simulink library "camera_update_lib"  (R2016b)
settings: Solver=ode45  StartTime=0.0  StopTime=10.0  RelTol=1e-3  EnableMultiTasking=on
undefined symbols (not defined in the file): accel_bias, ase_aug_state_bitmask, ase_hr_distance_r, ase_hr_r_mag, ase_local_mode_docking, ase_local_mode_map, ase_local_mode_perching, ase_minumum_resid_thresh, ase_ml_num_features, ase_of_num_aug, ase_of_num_features, ase_status_converged, ase_total_num_states, gyro_bias, hr_P_hr_ISS_ISS, hr_quat_ISS2hr, kfl_status, ml_mahal_distance, ml_P_cam_ISS_ISS, ml_quat_ISS2cam, of_mahal_distance, of_P_cam_ISS_ISS, of_quat_ISS2cam, P_EST_ISS_ISS, quat_ISS2B, tun_abp_q_body2dockcam, tun_abp_q_body2navcam, tun_abp_q_body2perchcam, tun_ase_dock_r_mag, tun_ase_dockcam_distortion, tun_ase_dockcam_inv_focal_length, tun_ase_enable_of, tun_ase_mahal_distance_max, tun_ase_map_error, tun_ase_min_hr_meas, tun_ase_min_ml_meas, tun_ase_min_of_meas, tun_ase_ml_forward_projection_time, tun_ase_navcam_distortion, tun_ase_navcam_inv_focal_length, tun_ase_of_r_mag, tun_ase_vis_r_mag, tun_ase_vocam_inv_focal_length, update_ML_features_cnt, update_OF_tracks_cnt, V_B_ISS_ISS
libraries: simulink x13, camera_update_lib x1
(part 1 of 2)
settings Model: Creator=jfusco1  LastModifiedBy=jfusco1
settings DataIOCC: LimitDataPoints=on  SaveFormat=Array
settings OptimizationCC: LifeSpan=inf
settings DebuggingCC: AllowSymbolicDim=off  SFUnexpectedBacktrackingDiag=warning  SFNoUnconditionalDefaultTransitionDiag=warning  SFExecutionAtInitializationDiag=none
settings HardwareCC: ProdBitPerPointer=32  ProdBitPerSizeT=32  ProdBitPerPtrDiffT=32  ProdLargestAtomicFloat=None  ProdIntDivRoundTo=Undefined  ProdEndianess=Unspecified  ProdWordSize=32  ProdHWDeviceType=32-bit Generic
settings ModelReferenceCC: PropagateSignalLabelsOutOfModel=off
settings GRTTargetCC: TargetLangStandard=C89/C90 (ANSI)  GeneratePreprocessorConditionals=Disable all
settings ConfigComp: CovMetricSettings=dw  CovHtmlReporting=on  CovSaveCumulativeToWorkspaceVar=on  CovSaveSingleToWorkspaceVar=on  CovExternalEMLEnable=off

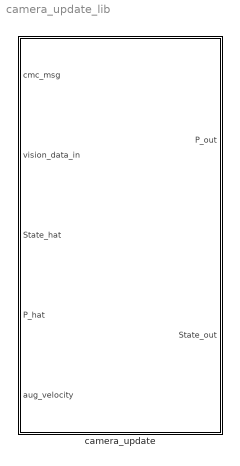
== system camera_update_lib ==
  camera_update : Subsystem

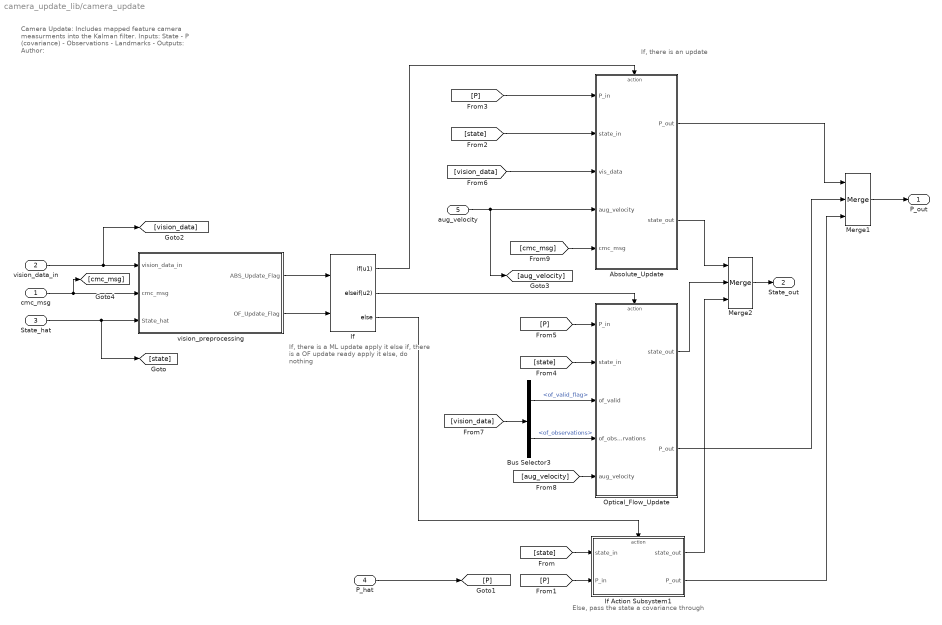
== system camera_update_lib/camera_update ==
  note: Camera Update:
      | Includes mapped feature camera measurments into the Kalman filter.
      |
      | Inputs:
      | State -
      | P (covariance) -
      | Observations -
      | Landmarks -
      |
      | Outputs:
      |
      | Author:
  note: If, there is an update
  note: Else, pass the state a covariance through
  note: If, there is a ML update apply it
      | else if, there is a OF update ready apply it
      | else, do nothing
  cmc_msg : Inport
  vision_data_in : Inport  Port=2
  State_hat : Inport  Port=3
  P_hat : Inport  Port=4  OutDataTypeStr=ase_cov_datatype
  aug_velocity : Inport  Port=5
  Absolute_Update : Subsystem  TreatAsAtomicUnit=on
  Bus Selector3 : BusSelector  OutputSignals=of_valid_flag,of_observations
  If : If  NumInputs=2  IfExpression=u1  ElseIfExpressions=u2
  If Action Subsystem1 : Subsystem  TreatAsAtomicUnit=on
  Merge1 : Merge  Inputs=3
  Merge2 : Merge  Inputs=3
  Optical_Flow_Update : Subsystem  TreatAsAtomicUnit=on
  vision_preprocessing : Subsystem
  P_out : Outport
  State_out : Outport  Port=2
  wires:
  cmc_msg/1 -> vision_preprocessing/2(cmc_msg), [cmc_msg]
  [aug_velocity] -> Optical_Flow_Update/5(aug_velocity)
  aug_velocity/1 -> Absolute_Update/4(aug_velocity), [aug_velocity]
  If/1 -> Absolute_Update/Action
  If/3 -> If Action Subsystem1/Action
  [P] -> If Action Subsystem1/2(P_in)
  [state] -> If Action Subsystem1/1(state_in)
  P_hat/1 -> [P]
  [state] -> Absolute_Update/2(state_in)
  [P] -> Absolute_Update/1(P_in)
  Absolute_Update/1(P_out) -> Merge1/1
  Merge1/1 -> P_out/1
  If Action Subsystem1/2(P_out) -> Merge1/3
  Merge2/1 -> State_out/1
  Absolute_Update/2(state_out) -> Merge2/1
  If Action Subsystem1/1(state_out) -> Merge2/3
  If/2 -> Optical_Flow_Update/Action
  [P] -> Optical_Flow_Update/1(P_in)
  [state] -> Optical_Flow_Update/2(state_in)
  [vision_data] -> Bus Selector3/1
  Bus Selector3/2 -> Optical_Flow_Update/4(of_observations)  "<of_observations>"
  Bus Selector3/1 -> Optical_Flow_Update/3(of_valid)  "<of_valid_flag>"
  Optical_Flow_Update/2(P_out) -> Merge1/2
  Optical_Flow_Update/1(state_out) -> Merge2/2
  vision_preprocessing/1("ABS_Update_Flag ") -> If/1
  vision_preprocessing/2(OF_Update_Flag) -> If/2
  State_hat/1 -> [state], vision_preprocessing/3(State_hat)
  vision_data_in/1 -> [vision_data], vision_preprocessing/1(vision_data_in)
  [vision_data] -> Absolute_Update/3(vis_data)
  [cmc_msg] -> Absolute_Update/5(cmc_msg)

== system camera_update_lib/camera_update/Absolute_Update ==
  P_in : Inport
  state_in : Inport  Port=2
  vis_data : Inport  Port=3
  aug_velocity : Inport  Port=4
  cmc_msg : Inport  Port=5
  Action Port : ActionPort  PropagateVarSize=During execution
  ML Update : Subsystem
  P_out : Outport
  state_out : Outport  Port=2
  wires:
  aug_velocity/1 -> ML Update/4(aug_velocity)
  state_in/1 -> ML Update/1(state_in)
  vis_data/1 -> ML Update/2(vis_data)
  P_in/1 -> ML Update/3(P_in)
  ML Update/1(State_out) -> state_out/1
  ML Update/2(P_out) -> P_out/1
  cmc_msg/1 -> ML Update/5(cmc_msg)

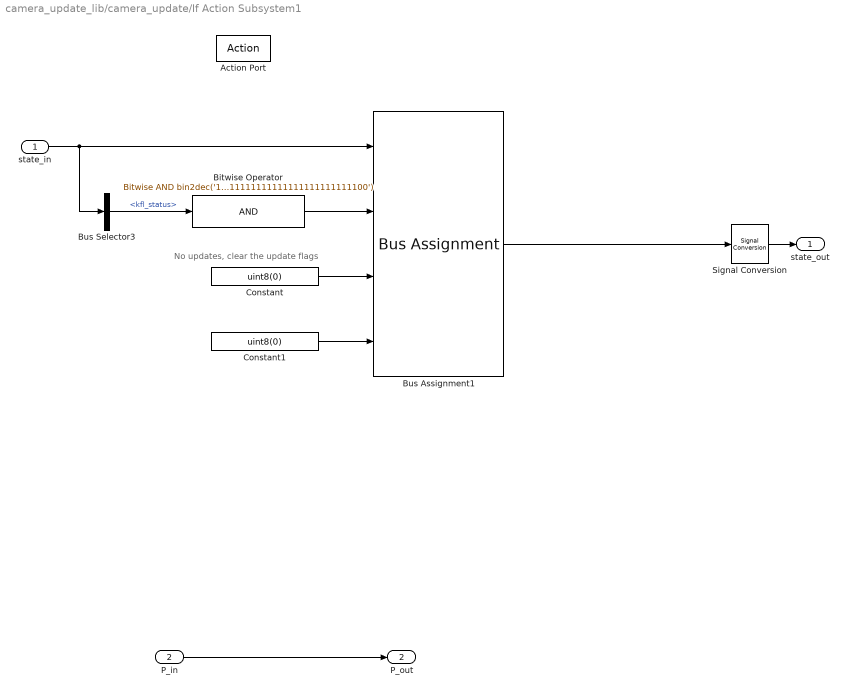
== system camera_update_lib/camera_update/If Action Subsystem1 ==
  note: No updates, clear the update flags
  state_in : Inport
  P_in : Inport  Port=2
  Action Port : ActionPort
  Bitwise Operator : simulink/Logic and Bit Operations/Bitwise Operator  logicop=AND  UseBitMask=on  BitMask=bin2dec('11111111111111111111111111111100')  BitMaskRealWorld=Stored Integer
  Bus Assignment1 : BusAssignment  AssignedSignals=kfl_status,update_OF_tracks_cnt,update_ML_features_cnt
  Bus Selector3 : BusSelector  OutputSignals=kfl_status
  Constant : Constant  Value=uint8(0)
  Constant1 : Constant  Value=uint8(0)
  Signal Conversion : SignalConversion  OverrideOpt=off
  state_out : Outport
  P_out : Outport  Port=2
  wires:
  Signal Conversion/1 -> state_out/1
  P_in/1 -> P_out/1
  Bus Selector3/1 -> Bitwise Operator/1  "<kfl_status>"
  Bitwise Operator/1 -> Bus Assignment1/2
  Bus Assignment1/1 -> Signal Conversion/1
  state_in/1 -> Bus Selector3/1, Bus Assignment1/1
  Constant/1 -> Bus Assignment1/3
  Constant1/1 -> Bus Assignment1/4

== system camera_update_lib/camera_update/Optical_Flow_Update ==
  P_in : Inport
  state_in : Inport  Port=2
  of_valid : Inport  Port=3
  of_observations : Inport  Port=4
  aug_velocity : Inport  Port=5
  Action Port : ActionPort  PropagateVarSize=During execution
  OF Update : Subsystem
  state_out : Outport
  P_out : Outport  Port=2
  wires:
  aug_velocity/1 -> OF Update/5(aug_velocity)
  OF Update/2(P_out) -> P_out/1
  OF Update/1(State_out) -> state_out/1
  P_in/1 -> OF Update/4(P_in)
  of_observations/1 -> OF Update/3(of_observations)
  of_valid/1 -> OF Update/2(of_valid)
  state_in/1 -> OF Update/1(state_in)

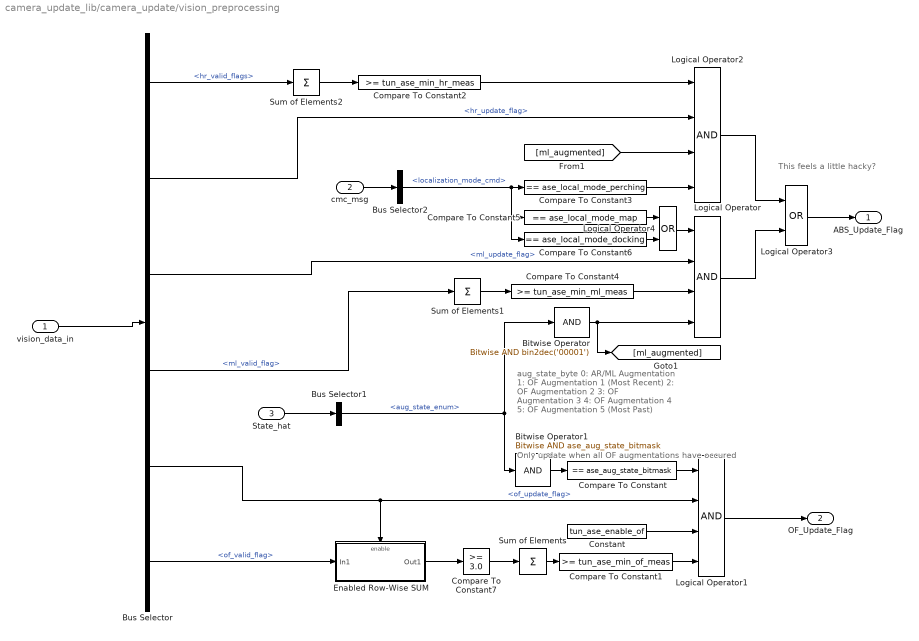
== system camera_update_lib/camera_update/vision_preprocessing ==
  note: This feels a little hacky?
  note: aug_state_byte
      | 0: AR/ML Augmentation
      | 1: OF Augmentation 1 (Most Recent)
      | 2: OF Augmentation 2
      | 3: OF Augmentation 3
      | 4: OF Augmentation 4
      | 5: OF Augmentation 5 (Most Past)
  note: Only update when all OF augmentations have occured
  vision_data_in : Inport
  cmc_msg : Inport  Port=2
  State_hat : Inport  Port=3
  Bitwise Operator : simulink/Logic and Bit Operations/Bitwise Operator  logicop=AND  UseBitMask=on  BitMask=bin2dec('00001')  BitMaskRealWorld=Stored Integer
  Bitwise Operator1 : simulink/Logic and Bit Operations/Bitwise Operator  logicop=AND  UseBitMask=on  BitMask=ase_aug_state_bitmask  BitMaskRealWorld=Stored Integer
  Bus Selector : BusSelector  OutputSignals=hr_valid_flags,hr_update_flag,ml_update_flag,ml_valid_flag,of_update_flag,of_valid_flag
  Bus Selector1 : BusSelector  OutputSignals=aug_state_enum
  Bus Selector2 : BusSelector  OutputSignals=localization_mode_cmd
  Compare To Constant : simulink/Logic and Bit Operations/Compare To Constant  relop===  const=ase_aug_state_bitmask  OutDataTypeStr=boolean
  Compare To Constant1 : simulink/Logic and Bit Operations/Compare To Constant  relop=>=  const=tun_ase_min_of_meas  OutDataTypeStr=boolean
  Compare To Constant2 : simulink/Logic and Bit Operations/Compare To Constant  relop=>=  const=tun_ase_min_hr_meas  OutDataTypeStr=boolean
  Compare To Constant3 : simulink/Logic and Bit Operations/Compare To Constant  relop===  const=ase_local_mode_perching  OutDataTypeStr=boolean
  Compare To Constant4 : simulink/Logic and Bit Operations/Compare To Constant  relop=>=  const=tun_ase_min_ml_meas  OutDataTypeStr=boolean
  Compare To Constant5 : simulink/Logic and Bit Operations/Compare To Constant  relop===  const=ase_local_mode_map  OutDataTypeStr=boolean
  Compare To Constant6 : simulink/Logic and Bit Operations/Compare To Constant  relop===  const=ase_local_mode_docking  OutDataTypeStr=boolean
  Compare To Constant7 : simulink/Logic and Bit Operations/Compare To Constant  relop=>=  const=3.0  OutDataTypeStr=boolean
  Constant : Constant  Value=tun_ase_enable_of
  Enabled Row-Wise SUM : Subsystem  TreatAsAtomicUnit=on
  Logical Operator : Logic  Inputs=4  AllPortsSameDT=off  OutDataTypeStr=boolean
  Logical Operator1 : Logic  Inputs=4  AllPortsSameDT=off  OutDataTypeStr=boolean
  Logical Operator2 : Logic  Inputs=4  AllPortsSameDT=off  OutDataTypeStr=boolean
  Logical Operator3 : Logic  Operator=OR  AllPortsSameDT=off  OutDataTypeStr=boolean
  Logical Operator4 : Logic  Operator=OR  AllPortsSameDT=off  OutDataTypeStr=boolean
  Sum of Elements : Sum  Inputs=+
  Sum of Elements1 : Sum  Inputs=+
  Sum of Elements2 : Sum  Inputs=+
  "ABS_Update_Flag " : Outport
  OF_Update_Flag : Outport  Port=2
  wires:
  Logical Operator3/1 -> "ABS_Update_Flag "/1
  Logical Operator/1 -> Logical Operator3/2
  Logical Operator2/1 -> Logical Operator3/1
  Bus Selector2/1 -> Compare To Constant3/1, Compare To Constant6/1, Compare To Constant5/1  "<localization_mode_cmd>"
  Compare To Constant3/1 -> Logical Operator2/4
  cmc_msg/1 -> Bus Selector2/1
  [ml_augmented] -> Logical Operator2/3
  Compare To Constant2/1 -> Logical Operator2/1
  Bus Selector/2 -> Logical Operator2/2  "<hr_update_flag>"
  Sum of Elements2/1 -> Compare To Constant2/1
  Bus Selector/1 -> Sum of Elements2/1  "<hr_valid_flags>"
  State_hat/1 -> Bus Selector1/1
  vision_data_in/1 -> Bus Selector/1
  Bus Selector/3 -> Logical Operator/2  "<ml_update_flag>"
  Bus Selector1/1 -> Bitwise Operator1/1, Bitwise Operator/1  "<aug_state_enum>"
  Bus Selector/5 -> Logical Operator1/2, Enabled Row-Wise SUM/Enable  "<of_update_flag>"
  Logical Operator1/1 -> OF_Update_Flag/1
  Constant/1 -> Logical Operator1/3
  Compare To Constant/1 -> Logical Operator1/1
  Bitwise Operator1/1 -> Compare To Constant/1
  Compare To Constant7/1 -> Sum of Elements/1
  Sum of Elements/1 -> Compare To Constant1/1
  Compare To Constant1/1 -> Logical Operator1/4
  Bitwise Operator/1 -> Logical Operator/4, [ml_augmented]
  Compare To Constant4/1 -> Logical Operator/3
  Sum of Elements1/1 -> Compare To Constant4/1
  Bus Selector/4 -> Sum of Elements1/1  "<ml_valid_flag>"
  Compare To Constant5/1 -> Logical Operator4/1
  Compare To Constant6/1 -> Logical Operator4/2
  Logical Operator4/1 -> Logical Operator/1
  Bus Selector/6 -> Enabled Row-Wise SUM/1(In1)  "<of_valid_flag>"
  Enabled Row-Wise SUM/1(Out1) -> Compare To Constant7/1

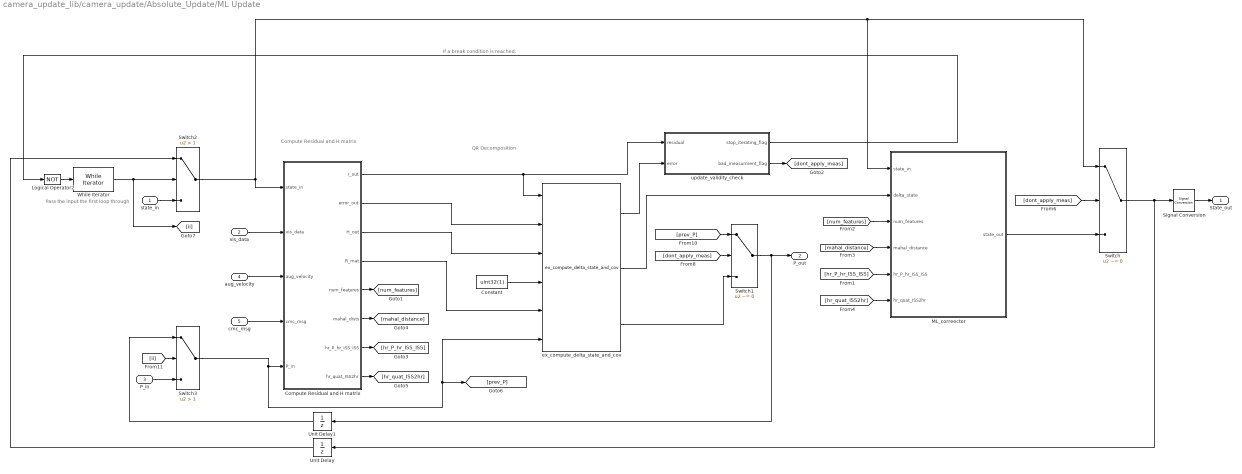
== system camera_update_lib/camera_update/Absolute_Update/ML Update ==
  note: Compute Residual and H matrix
  note: QR Decomposition
  note: Pass the input the first loop through
  note: If a break condition is reached.
  state_in : Inport
  vis_data : Inport  Port=2
  P_in : Inport  Port=3
  aug_velocity : Inport  Port=4
  cmc_msg : Inport  Port=5
  Compute Residual and H matrix : Subsystem
  Constant : Constant  Value=uint32(1)
  Logical Operator2 : Logic  Operator=NOT  Inputs=1  AllPortsSameDT=off  OutDataTypeStr=boolean
  ML_correector : Subsystem
  Signal Conversion : SignalConversion  OverrideOpt=off
  Switch : Switch  Criteria=u2 ~= 0
  Switch1 : Switch  Criteria=u2 ~= 0
  Switch2 : Switch  Criteria=u2 > Threshold  Threshold=1
  Switch3 : Switch  Criteria=u2 > Threshold  Threshold=1
  Unit Delay : UnitDelay  SampleTime=-1
  Unit Delay1 : UnitDelay  SampleTime=-1
  While Iterator : WhileIterator  MaxIters=ase_max_update_iterations  WhileBlockType=do-while  ResetStates=reset  ShowIterationPort=on
  ex_compute_delta_state_and_cov : S-Function  FunctionName=ex_compute_delta_state_and_cov  SFunctionDeploymentMode=off  EnableBusSupport=off  mask(Legacy Function){SFunctionSpec=int32 y1 = compute_delta_state_and_cov(single u1[], int32 u2, single u3[][], int32 size(u3, 1), int32 size(u3, 2),uint32 u4, single u5[][], single u6[][],single y2[size(u3, 2)], single y3[size(u3, 2)][size(u3, 2)]), ShowSpec=off}
      mask prompts: ShowSpec "Display function specification"
      mask help:
      | This block allows you to call the legacy functions specified by the following Legacy Code Tool definition:
      | def.SFunctionName = 'ex_compute_delta_state_and_cov';
      | def.OutputFcnSpec = 'int32 y1 = compute_delta_state_and_cov(single u1[], int32 u2, single u3[][], int32 size(u3, 1), int32 size(u3, 2),uint32 u4, single u5[][], single u6[][],single y2[size(u3, 2)], single y3[size(u3, 2)][size(u3, 2)])';
      | def.HeaderFiles = {'compute_delta_state_and_cov.h'};
      | def.SourceFiles = {'compute_delta_state_and_cov.cpp'};
      | def.IncPaths = {'cxx_functions/include', '/usr/include/eigen3'};
      | def.SrcPaths = {'cxx_functions/src', '/usr/include/eigen3/Eigen/src'};
      | def.Options.language = 'C++';
      mask Help: <p>This block was generated automatically by the Legacy Code Tool. For detailed help on this tool, call<a href="matlab:legacy_code('help')"> legacy_code('help')</a>.</p>
      mask Callback ShowSpec:
      | if strcmp(get_param(gcbh, 'ShowSpec'), 'on')
      |   set_param(gcbh, 'MaskDisplay', sprintf('fprintf(''%s'');', get_param(gcbh, 'SFunctionSpec')));
      | else
      |   set_param(gcbh, 'MaskDisplay', sprintf('fprintf(''%s'');', get_param(gcbh, 'FunctionName')));
      | end
      mask Display: fprintf('ex_compute_delta_state_and_cov');
  update_validity_check : Subsystem
  State_out : Outport
  P_out : Outport  Port=2
  wires:
  ex_compute_delta_state_and_cov/2 -> ML_correector/2(delta_state)
  ex_compute_delta_state_and_cov/3 -> Switch1/3
  Compute Residual and H matrix/3(H_out) -> ex_compute_delta_state_and_cov/3
  Compute Residual and H matrix/1(r_out) -> ex_compute_delta_state_and_cov/1, update_validity_check/1(residual)
  update_validity_check/2(bad_measurment_flag) -> [dont_apply_meas]
  [prev_P] -> Switch1/1
  Switch1/1 -> P_out/1, Unit Delay1/1
  [dont_apply_meas] -> Switch1/2
  Switch2/1 -> ML_correector/1(state_in), Switch/1, Compute Residual and H matrix/1(state_in)
  Switch/1 -> Unit Delay/1, Signal Conversion/1
  [dont_apply_meas] -> Switch/2
  Compute Residual and H matrix/4(R_mat) -> ex_compute_delta_state_and_cov/5
  Signal Conversion/1 -> State_out/1
  Switch3/1 -> Compute Residual and H matrix/5(P_in), ex_compute_delta_state_and_cov/6, [prev_P]
  state_in/1 -> Switch2/3
  Unit Delay/1 -> Switch2/1
  P_in/1 -> Switch3/3
  Unit Delay1/1 -> Switch3/1
  While Iterator/1 -> [ii], Switch2/2
  [ii] -> Switch3/2
  Logical Operator2/1 -> While Iterator/1
  update_validity_check/1(stop_iterating_flag) -> Logical Operator2/1
  ML_correector/1(state_out) -> Switch/3
  Compute Residual and H matrix/2(error_out) -> ex_compute_delta_state_and_cov/2
  Compute Residual and H matrix/5(num_features) -> [num_features]
  Compute Residual and H matrix/6(mahal_dists) -> [mahal_distance]
  vis_data/1 -> Compute Residual and H matrix/2(vis_data)
  ex_compute_delta_state_and_cov/1 -> update_validity_check/2(error)
  [num_features] -> ML_correector/3(num_features)
  [mahal_distance] -> ML_correector/4(mahal_distance)
  aug_velocity/1 -> Compute Residual and H matrix/3(aug_velocity)
  cmc_msg/1 -> Compute Residual and H matrix/4(cmc_msg)
  [hr_quat_ISS2hr] -> ML_correector/6(hr_quat_ISS2hr)
  [hr_P_hr_ISS_ISS] -> ML_correector/5(hr_P_hr_ISS_ISS)
  Compute Residual and H matrix/7(hr_P_hr_ISS_ISS) -> [hr_P_hr_ISS_ISS]
  Compute Residual and H matrix/8(hr_quat_ISS2hr) -> [hr_quat_ISS2hr]
  Constant/1 -> ex_compute_delta_state_and_cov/4

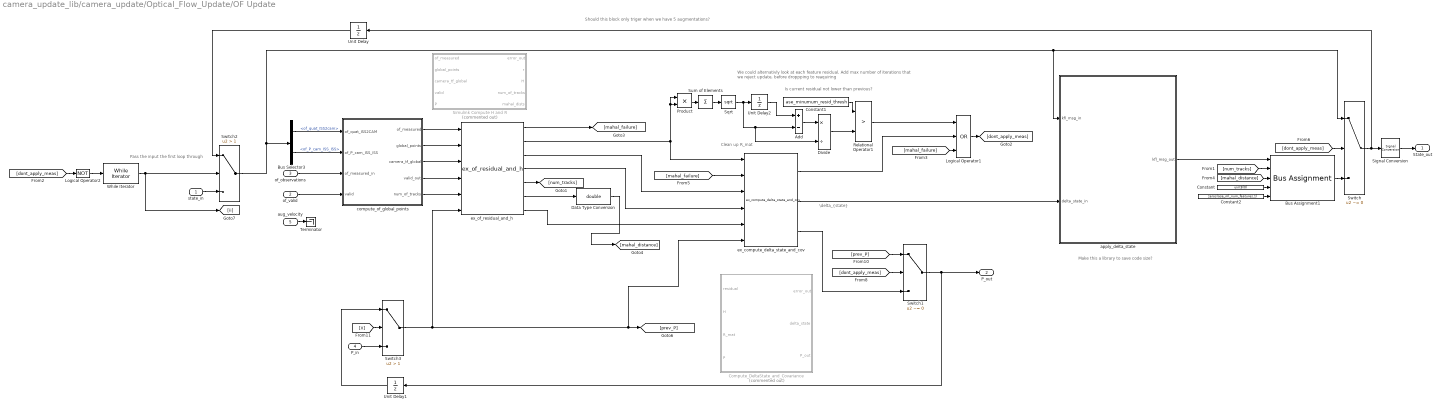
== system camera_update_lib/camera_update/Optical_Flow_Update/OF Update ==
  note: Clean up R_mat
  note: Pass the input the first loop through
  note: \delta_{state}
  note: Make this a library to save code size?
  note: Should this block only triger when we have 5 augmentations?
  note: Is current residual not lower than previous?
  note: We could alternativly look at each feature residual.
      | Add max number of iterations that we reject update, before droppping to reaquiring
  state_in : Inport
  of_valid : Inport  Port=2
  of_observations : Inport  Port=3
  P_in : Inport  Port=4  PortDimensions=[ase_total_num_states ase_total_num_states]
  aug_velocity : Inport  Port=5
  Add : Sum  Inputs=+-
  Bus Assignment1 : BusAssignment  AssignedSignals=update_OF_tracks_cnt,of_mahal_distance,update_ML_features_cnt,ml_mahal_distance
  Bus Selector3 : BusSelector  OutputSignals=of_quat_ISS2cam,of_P_cam_ISS_ISS
  Compute_DeltaState_and_Covariance : MATLAB Function  Commented=on  TreatAsAtomicUnit=on
  Constant : Constant  Value=uint8(0)
  Constant1 : Constant  Value=ase_minumum_resid_thresh
  Constant2 : Constant  Value=zeros(ase_ml_num_features,1)
  Data Type Conversion : DataTypeConversion  OutDataTypeStr=double
  Divide : Product  Inputs=*/
  Logical Operator1 : Logic  Operator=OR  Inputs=3  AllPortsSameDT=off  OutDataTypeStr=boolean
  Logical Operator2 : Logic  Operator=NOT  Inputs=1  AllPortsSameDT=off  OutDataTypeStr=boolean
  Product : Product
  Relational Operator1 : RelationalOperator  Operator=>  OutDataTypeStr=boolean  RndMeth=Nearest
  Signal Conversion : SignalConversion  OverrideOpt=off
  Simulink Compute H and R : Subsystem  Commented=on  TreatAsAtomicUnit=on
  Sqrt : Sqrt  SaturateOnIntegerOverflow=on
  Sum of Elements : Sum  Inputs=+
  Switch : Switch  Criteria=u2 ~= 0
  Switch1 : Switch  Criteria=u2 ~= 0
  Switch2 : Switch  Criteria=u2 > Threshold  Threshold=1
  Switch3 : Switch  Criteria=u2 > Threshold  Threshold=1
  Terminator : Terminator
  Unit Delay : UnitDelay  SampleTime=-1
  Unit Delay1 : UnitDelay  SampleTime=-1
  Unit Delay2 : UnitDelay  InitialCondition=inf  SampleTime=-1
      settings: AttributesFormatString=IC: %<InitialCondition>
  While Iterator : WhileIterator  MaxIters=ase_max_of_update_iterations  WhileBlockType=do-while  ResetStates=reset  ShowIterationPort=on
  apply_delta_state : Subsystem
  compute_of_global_points : MATLAB Function  TreatAsAtomicUnit=on
  ex_compute_delta_state_and_cov : S-Function  FunctionName=ex_compute_delta_state_and_cov  SFunctionDeploymentMode=off  EnableBusSupport=off  mask(Legacy Function){SFunctionSpec=int32 y1 = compute_delta_state_and_cov(single u1[], int32 u2, single u3[][], int32 size(u3, 1), int32 size(u3, 2),uint32 u4, single u5[][], single u6[][],single y2[size(u3, 2)], single y3[size(u3, 2)][size(u3, 2)]), ShowSpec=off}
      mask prompts: ShowSpec "Display function specification"
      mask help:
      | This block allows you to call the legacy functions specified by the following Legacy Code Tool definition:
      | def.SFunctionName = 'ex_compute_delta_state_and_cov';
      | def.OutputFcnSpec = 'int32 y1 = compute_delta_state_and_cov(single u1[], int32 u2, single u3[][], int32 size(u3, 1), int32 size(u3, 2),uint32 u4, single u5[][], single u6[][],single y2[size(u3, 2)], single y3[size(u3, 2)][size(u3, 2)])';
      | def.HeaderFiles = {'compute_delta_state_and_cov.h'};
      | def.SourceFiles = {'compute_delta_state_and_cov.cpp'};
      | def.IncPaths = {'cxx_functions/include', '/usr/include/eigen3'};
      | def.SrcPaths = {'cxx_functions/src', '/usr/include/eigen3/Eigen/src'};
      | def.Options.language = 'C++';
      mask Help: <p>This block was generated automatically by the Legacy Code Tool. For detailed help on this tool, call<a href="matlab:legacy_code('help')"> legacy_code('help')</a>.</p>
      mask Callback ShowSpec:
      | if strcmp(get_param(gcbh, 'ShowSpec'), 'on')
      |   set_param(gcbh, 'MaskDisplay', sprintf('fprintf(''%s'');', get_param(gcbh, 'SFunctionSpec')));
      | else
      |   set_param(gcbh, 'MaskDisplay', sprintf('fprintf(''%s'');', get_param(gcbh, 'FunctionName')));
      | end
      mask Display: fprintf('ex_compute_delta_state_and_cov');
  ex_of_residual_and_h : S-Function  FunctionName=ex_of_residual_and_h  Parameters=SParameter1, SParameter2, SParameter3, SParameter4, SParameter5, SParameter6  SFunctionDeploymentMode=off  EnableBusSupport=off  mask(Legacy Function){SFunctionSpec=int32 y1 = of_residual_and_h(single u1[1600], single u2[4][50], single u3[64][4], int32 u4[50][16], int32 u5, int32 p1, int32 p2, single p3, single p4, single p5, single p6, single u6[117][117], single y2[96], single y3[96][117], uint32 y4[1], uint8 y5[1], single y6[50], single y7[96][96]), SParameter1=ase_of_num_aug, SParameter2=ase_of_num_features, SParameter3=tun_ase_mahal_distance_max, SParameter4=tun_ase_of_r_mag, SParameter5=tun_ase_navcam_inv_focal_length, SParameter6=tun_ase_navcam_distortion, ShowSpec=off}
      mask prompts: SParameter1 "P1:"; SParameter2 "P2:"; SParameter3 "P3:"; SParameter4 "P4:"; SParameter5 "P5:"; SParameter6 "P6:"; ShowSpec "Display function specification"
      mask help:
      | This block allows you to call the legacy functions specified by the following Legacy Code Tool definition:
      | def.SFunctionName = 'ex_of_residual_and_h';
      | def.OutputFcnSpec = 'int32 y1 = of_residual_and_h(single u1[1600], single u2[4][50], single u3[64][4], int32 u4[50][16], int32 u5, int32 p1, int32 p2, single p3, single p4, single p5, single p6, single u6[117][117], single y2[96], single y3[96][117], uint32 y4[1], uint8 y5[1], single y6[50], single y7[96][96])';
      | def.HeaderFiles = {'of_residual_and_h.h'};
      | def.SourceFiles = {'of_residual_and_h.cpp'};
      | def.IncPaths = {'./cxx_functions/include', '/usr/include/eigen3/'};
      | def.SrcPaths = {'./cxx_functions/src', '/usr/include/eigen3/Eigen/src'};
      | def.Options.language = 'C++';
      | def.Options.supportsMultipleExecInstances = true;
      mask Help: <p>This block was generated automatically by the Legacy Code Tool. For detailed help on this tool, call<a href="matlab:legacy_code('help')"> legacy_code('help')</a>.</p>
      mask Callback ShowSpec:
      | if strcmp(get_param(gcbh, 'ShowSpec'), 'on')
      |   set_param(gcbh, 'MaskDisplay', sprintf('fprintf(''%s'');', get_param(gcbh, 'SFunctionSpec')));
      | else
      |   set_param(gcbh, 'MaskDisplay', sprintf('fprintf(''%s'');', get_param(gcbh, 'FunctionName')));
      | end
      mask Display: fprintf('ex_of_residual_and_h');
  State_out : Outport
  P_out : Outport  Port=2
  wires:
  Constant2/1 -> Bus Assignment1/5
  Constant/1 -> Bus Assignment1/4
  [mahal_distance] -> Bus Assignment1/3
  Logical Operator2/1 -> While Iterator/1
  [ii] -> Switch3/2
  While Iterator/1 -> Switch2/2, [ii]
  Unit Delay1/1 -> Switch3/1
  P_in/1 -> Switch3/3
  Unit Delay/1 -> Switch2/1
  state_in/1 -> Switch2/3
  Switch3/1 -> ex_of_residual_and_h/6, ex_compute_delta_state_and_cov/6, [prev_P]
  Signal Conversion/1 -> State_out/1
  [dont_apply_meas] -> Switch/2
  Switch/1 -> Unit Delay/1, Signal Conversion/1
  Switch2/1 -> apply_delta_state/1(kfl_msg_in), Switch/1, Bus Selector3/1
  [dont_apply_meas] -> Switch1/2
  Switch1/1 -> P_out/1, Unit Delay1/1
  [prev_P] -> Switch1/1
  Bus Selector3/1 -> compute_of_global_points/1(of_quat_ISS2CAM)  "<of_quat_ISS2cam>"
  Bus Selector3/2 -> compute_of_global_points/2(of_P_cam_ISS_ISS)  "<of_P_cam_ISS_ISS>"
  of_valid/1 -> compute_of_global_points/4(valid)
  of_observations/1 -> compute_of_global_points/3(of_measured_in)
  [num_tracks] -> Bus Assignment1/2
  Bus Assignment1/1 -> Switch/3
  aug_velocity/1 -> Terminator/1
  Constant1/1 -> Relational Operator1/1
  Divide/1 -> Relational Operator1/2
  Add/1 -> Divide/1
  Product/1 -> Sum of Elements/1
  Unit Delay2/1 -> Add/1
  ex_of_residual_and_h/2 -> ex_compute_delta_state_and_cov/1, Product/1, Product/2
  Sqrt/1 -> Divide/2, Add/2, Unit Delay2/1
  Logical Operator1/1 -> [dont_apply_meas]
  Relational Operator1/1 -> Logical Operator1/1
  [dont_apply_meas] -> Logical Operator2/1
  ex_of_residual_and_h/1 -> [mahal_failure]
  ex_of_residual_and_h/5 -> [num_tracks]
  Data Type Conversion/1 -> [mahal_distance]
  ex_of_residual_and_h/6 -> Data Type Conversion/1
  compute_of_global_points/5(num_of_tracks) -> ex_of_residual_and_h/5
  compute_of_global_points/4(valid_out) -> ex_of_residual_and_h/4
  compute_of_global_points/3(camera_tf_global) -> ex_of_residual_and_h/3
  compute_of_global_points/2(global_points) -> ex_of_residual_and_h/2
  compute_of_global_points/1(of_measured) -> ex_of_residual_and_h/1
  [mahal_failure] -> ex_compute_delta_state_and_cov/2
  ex_compute_delta_state_and_cov/1 -> Logical Operator1/2
  ex_compute_delta_state_and_cov/2 -> apply_delta_state/2(delta_state_in)
  ex_compute_delta_state_and_cov/3 -> Switch1/3
  ex_of_residual_and_h/3 -> ex_compute_delta_state_and_cov/3
  ex_of_residual_and_h/4 -> ex_compute_delta_state_and_cov/4
  Sum of Elements/1 -> Sqrt/1
  [mahal_failure] -> Logical Operator1/3
  apply_delta_state/1(kfl_msg_out) -> Bus Assignment1/1
  ex_of_residual_and_h/7 -> ex_compute_delta_state_and_cov/5

== system camera_update_lib/camera_update/vision_preprocessing/Enabled Row-Wise SUM ==
  In1 : Inport
  Enable : EnablePort
  Sum of Elements3 : Sum  Inputs=+  CollapseMode=Specified dimension  CollapseDim=2
  Out1 : Outport
  wires:
  In1/1 -> Sum of Elements3/1
  Sum of Elements3/1 -> Out1/1

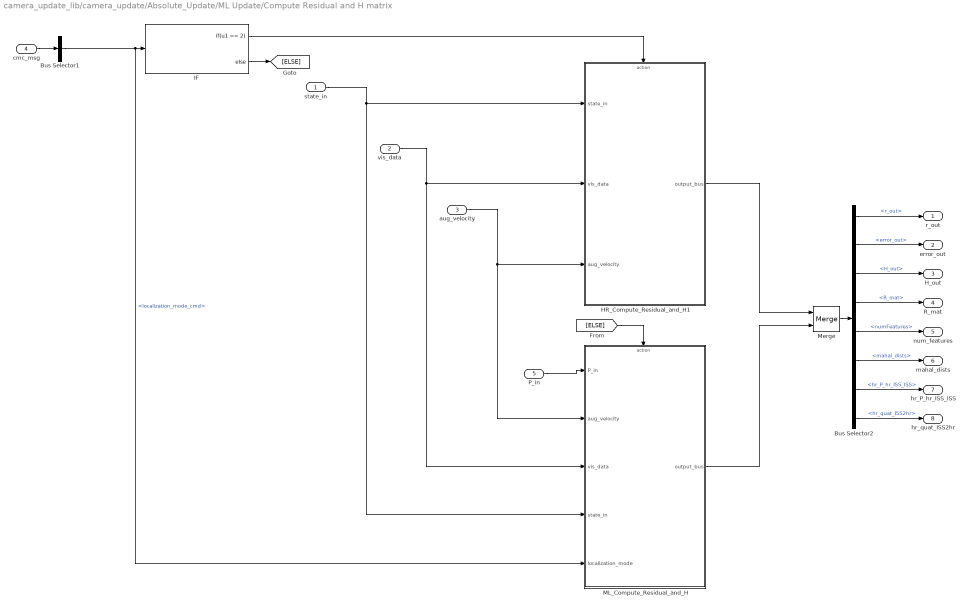
== system camera_update_lib/camera_update/Absolute_Update/ML Update/Compute Residual and H matrix ==
  state_in : Inport
  vis_data : Inport  Port=2
  aug_velocity : Inport  Port=3
  cmc_msg : Inport  Port=4
  P_in : Inport  Port=5
  Bus Selector1 : BusSelector  OutputSignals=localization_mode_cmd
  Bus Selector2 : BusSelector  OutputSignals=r_out,error_out,H_out,R_mat,numFeatures,mahal_dists,hr_P_hr_ISS_ISS,hr_quat_ISS2hr
  HR_Compute_Residual_and_H1 : Subsystem  TreatAsAtomicUnit=on
  IF : If  IfExpression=u1 == 2
  ML_Compute_Residual_and_H : Subsystem  TreatAsAtomicUnit=on
  Merge : Merge
  r_out : Outport
  error_out : Outport  Port=2
  H_out : Outport  Port=3
  R_mat : Outport  Port=4
  num_features : Outport  Port=5
  mahal_dists : Outport  Port=6
  hr_P_hr_ISS_ISS : Outport  Port=7
  hr_quat_ISS2hr : Outport  Port=8
  wires:
  IF/1 -> HR_Compute_Residual_and_H1/Action
  state_in/1 -> ML_Compute_Residual_and_H/4(state_in), HR_Compute_Residual_and_H1/1(state_in)
  vis_data/1 -> ML_Compute_Residual_and_H/3(vis_data), HR_Compute_Residual_and_H1/2(vis_data)
  P_in/1 -> ML_Compute_Residual_and_H/1(P_in)
  aug_velocity/1 -> ML_Compute_Residual_and_H/2(aug_velocity), HR_Compute_Residual_and_H1/3(aug_velocity)
  IF/2 -> [ELSE]
  [ELSE] -> ML_Compute_Residual_and_H/Action
  Merge/1 -> Bus Selector2/1
  Bus Selector2/1 -> r_out/1  "<r_out>"
  Bus Selector2/2 -> error_out/1  "<error_out>"
  Bus Selector2/3 -> H_out/1  "<H_out>"
  Bus Selector2/4 -> R_mat/1  "<R_mat>"
  Bus Selector2/5 -> num_features/1  "<numFeatures>"
  Bus Selector2/6 -> mahal_dists/1  "<mahal_dists>"
  HR_Compute_Residual_and_H1/1(output_bus) -> Merge/1
  ML_Compute_Residual_and_H/1(output_bus) -> Merge/2
  cmc_msg/1 -> Bus Selector1/1
  Bus Selector1/1 -> ML_Compute_Residual_and_H/5(localization_mode), IF/1  "<localization_mode_cmd>"
  Bus Selector2/7 -> hr_P_hr_ISS_ISS/1  "<hr_P_hr_ISS_ISS>"
  Bus Selector2/8 -> hr_quat_ISS2hr/1  "<hr_quat_ISS2hr>"

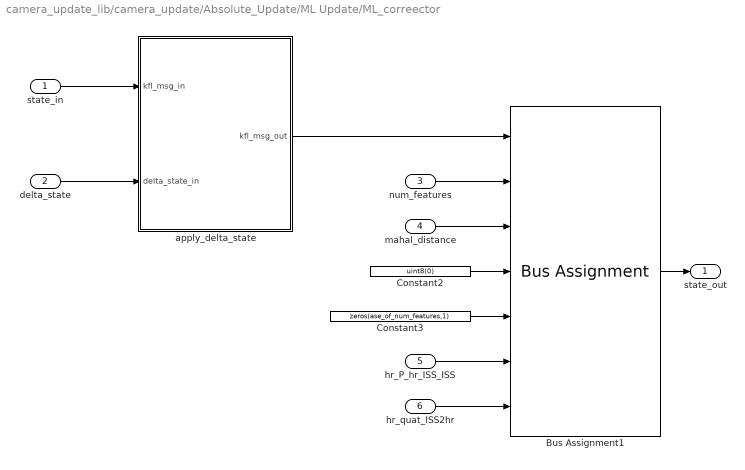
== system camera_update_lib/camera_update/Absolute_Update/ML Update/ML_correector ==
  state_in : Inport
  delta_state : Inport  Port=2
  num_features : Inport  Port=3
  mahal_distance : Inport  Port=4
  hr_P_hr_ISS_ISS : Inport  Port=5
  hr_quat_ISS2hr : Inport  Port=6
  Bus Assignment1 : BusAssignment  AssignedSignals=update_ML_features_cnt,ml_mahal_distance,update_OF_tracks_cnt,of_mahal_distance,hr_P_hr_ISS_ISS,hr_quat_ISS2hr
  Constant2 : Constant  Value=uint8(0)
  Constant3 : Constant  Value=zeros(ase_of_num_features,1)
  apply_delta_state : Subsystem
  state_out : Outport
  wires:
  mahal_distance/1 -> Bus Assignment1/3
  num_features/1 -> Bus Assignment1/2
  Constant2/1 -> Bus Assignment1/4
  Constant3/1 -> Bus Assignment1/5
  Bus Assignment1/1 -> state_out/1
  hr_quat_ISS2hr/1 -> Bus Assignment1/7
  hr_P_hr_ISS_ISS/1 -> Bus Assignment1/6
  apply_delta_state/1(kfl_msg_out) -> Bus Assignment1/1
  delta_state/1 -> apply_delta_state/2(delta_state_in)
  state_in/1 -> apply_delta_state/1(kfl_msg_in)

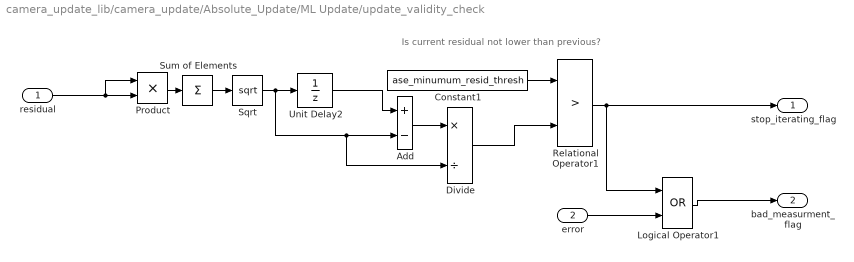
== system camera_update_lib/camera_update/Absolute_Update/ML Update/update_validity_check ==
  note: Is current residual not lower than previous?
  residual : Inport
  error : Inport  Port=2
  Add : Sum  Inputs=+-
  Constant1 : Constant  Value=ase_minumum_resid_thresh
  Divide : Product  Inputs=*/
  Logical Operator1 : Logic  Operator=OR  AllPortsSameDT=off  OutDataTypeStr=boolean
  Product : Product
  Relational Operator1 : RelationalOperator  Operator=>  OutDataTypeStr=boolean  RndMeth=Nearest
  Sqrt : Sqrt  SaturateOnIntegerOverflow=on
  Sum of Elements : Sum  Inputs=+
  Unit Delay2 : UnitDelay  InitialCondition=inf  SampleTime=-1
      settings: AttributesFormatString=IC: %<InitialCondition>
  stop_iterating_flag : Outport
  bad_measurment_flag : Outport  Port=2
  wires:
  residual/1 -> Product/2, Product/1
  Logical Operator1/1 -> bad_measurment_flag/1
  Unit Delay2/1 -> Add/1
  Product/1 -> Sum of Elements/1
  Sum of Elements/1 -> Sqrt/1
  Sqrt/1 -> Divide/2, Add/2, Unit Delay2/1
  Add/1 -> Divide/1
  Divide/1 -> Relational Operator1/2
  Constant1/1 -> Relational Operator1/1
  Relational Operator1/1 -> stop_iterating_flag/1, Logical Operator1/1
  error/1 -> Logical Operator1/2

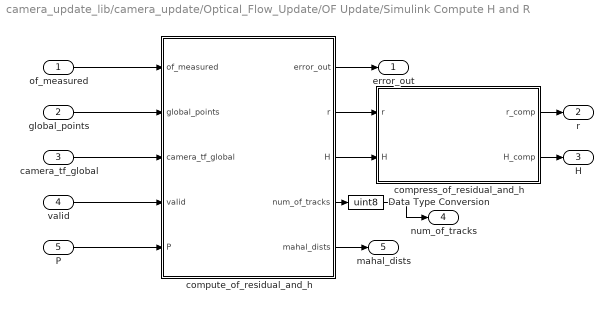
== system camera_update_lib/camera_update/Optical_Flow_Update/OF Update/Simulink Compute H and R ==
  of_measured : Inport
  global_points : Inport  Port=2
  camera_tf_global : Inport  Port=3
  valid : Inport  Port=4
  P : Inport  Port=5
  Data Type Conversion : DataTypeConversion  OutDataTypeStr=uint8
  compress_of_residual_and_h : MATLAB Function  TreatAsAtomicUnit=on
  compute_of_residual_and_h : MATLAB Function  TreatAsAtomicUnit=on
  error_out : Outport
  r : Outport  Port=2
  H : Outport  Port=3
  num_of_tracks : Outport  Port=4
  mahal_dists : Outport  Port=5
  wires:
  compute_of_residual_and_h/3(H) -> compress_of_residual_and_h/2(H)
  compute_of_residual_and_h/2(r) -> compress_of_residual_and_h/1(r)
  camera_tf_global/1 -> compute_of_residual_and_h/3(camera_tf_global)
  global_points/1 -> compute_of_residual_and_h/2(global_points)
  of_measured/1 -> compute_of_residual_and_h/1(of_measured)
  compress_of_residual_and_h/1(r_comp) -> r/1
  compute_of_residual_and_h/4(num_of_tracks) -> Data Type Conversion/1
  valid/1 -> compute_of_residual_and_h/4(valid)
  P/1 -> compute_of_residual_and_h/5(P)
  compress_of_residual_and_h/2(H_comp) -> H/1
  Data Type Conversion/1 -> num_of_tracks/1
  compute_of_residual_and_h/5(mahal_dists) -> mahal_dists/1
  compute_of_residual_and_h/1(error_out) -> error_out/1

== system camera_update_lib/camera_update/Optical_Flow_Update/OF Update/apply_delta_state ==
  kfl_msg_in : Inport
  delta_state_in : Inport  Port=2
  Bus Assignment1 : BusAssignment  AssignedSignals=quat_ISS2B,gyro_bias,V_B_ISS_ISS,accel_bias,P_EST_ISS_ISS,ml_quat_ISS2cam,ml_P_cam_ISS_ISS,kfl_status,of_quat_ISS2cam,of_P_cam_ISS_ISS
  Bus Selector1 : BusSelector  OutputSignals=quat_ISS2B,gyro_bias,V_B_ISS_ISS,accel_bias,P_EST_ISS_ISS,ml_quat_ISS2cam,ml_P_cam_ISS_ISS,kfl_status,of_quat_ISS2cam,of_P_cam_ISS_ISS
  Constant : Constant  Value=uint16(2)
  ex_apply_delta_state : camera_update_lib/camera_update/Absolute_Update/ML Update/ML_correector/apply_delta_state/ex_apply_delta_state  SFunctionSpec=void apply_delta_state(single u1[], int32 size(u1, 1), uint16 u2, single u3[4], single u4[3], single u5[3], single u6[3], single u7[3], single u8[4], single u9[3], uint16 u10, single u11[16][4], single u12[16][3], single y1[4], single y2[3], single y3[3], single y4[3], single y5[3], single y6[4], single y7[3], uint16 y8[1], single y9[16][4], single y10[16][3])  ShowSpec=off
  kfl_msg_out : Outport  OutDataTypeStr=Bus: kfl_msg
  wires:
  ex_apply_delta_state/10 -> Bus Assignment1/11
  ex_apply_delta_state/8 -> Bus Assignment1/9
  ex_apply_delta_state/7 -> Bus Assignment1/8
  ex_apply_delta_state/5 -> Bus Assignment1/6
  ex_apply_delta_state/4 -> Bus Assignment1/5
  ex_apply_delta_state/3 -> Bus Assignment1/4
  ex_apply_delta_state/2 -> Bus Assignment1/3
  Bus Selector1/10 -> ex_apply_delta_state/12  "<of_P_cam_ISS_ISS>"
  Bus Selector1/9 -> ex_apply_delta_state/11  "<of_quat_ISS2cam>"
  Bus Selector1/8 -> ex_apply_delta_state/10  "<kfl_status>"
  Bus Selector1/7 -> ex_apply_delta_state/9  "<ml_P_cam_ISS_ISS>"
  Bus Selector1/6 -> ex_apply_delta_state/8  "<ml_quat_ISS2cam>"
  Bus Selector1/5 -> ex_apply_delta_state/7  "<P_EST_ISS_ISS>"
  Bus Selector1/4 -> ex_apply_delta_state/6  "<accel_bias>"
  Bus Selector1/3 -> ex_apply_delta_state/5  "<V_B_ISS_ISS>"
  Bus Selector1/2 -> ex_apply_delta_state/4  "<gyro_bias>"
  Bus Selector1/1 -> ex_apply_delta_state/3  "<quat_ISS2B>"
  Constant/1 -> ex_apply_delta_state/2
  delta_state_in/1 -> ex_apply_delta_state/1
  kfl_msg_in/1 -> Bus Assignment1/1, Bus Selector1/1
  Bus Assignment1/1 -> kfl_msg_out/1
  ex_apply_delta_state/1 -> Bus Assignment1/2
  ex_apply_delta_state/9 -> Bus Assignment1/10
  ex_apply_delta_state/6 -> Bus Assignment1/7

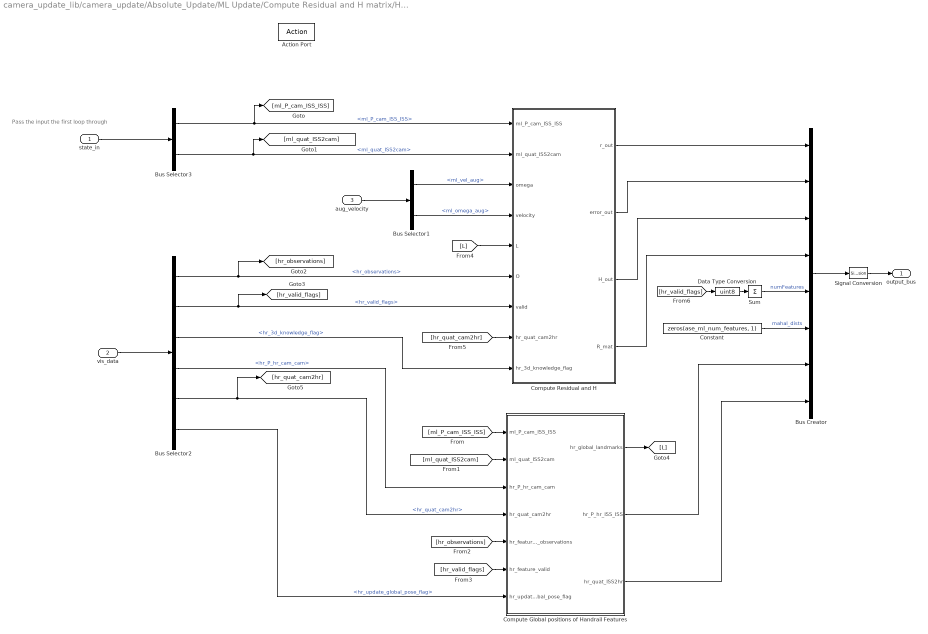
== system camera_update_lib/camera_update/Absolute_Update/ML Update/Compute Residual and H matrix/HR_Compute_Residual_and_H1 ==
  note: Pass the input the first loop through
  state_in : Inport
  vis_data : Inport  Port=2
  aug_velocity : Inport  Port=3
  Action Port : ActionPort
  Bus Creator : BusCreator  Inputs=8
  Bus Selector1 : BusSelector  OutputSignals=ml_vel_aug,ml_omega_aug
  Bus Selector2 : BusSelector  OutputSignals=hr_observations,hr_valid_flags,hr_3d_knowledge_flag,hr_P_hr_cam_cam,hr_quat_cam2hr,hr_update_global_pose_flag
  Bus Selector3 : BusSelector  OutputSignals=ml_P_cam_ISS_ISS,ml_quat_ISS2cam
  Compute Global positions of Handrail Features : MATLAB Function  TreatAsAtomicUnit=on
  Compute Residual and H : MATLAB Function  TreatAsAtomicUnit=on
  Constant : Constant  Value=zeros(ase_ml_num_features, 1)  VectorParams1D=off
  Data Type Conversion : DataTypeConversion  OutDataTypeStr=uint8
  Signal Conversion : SignalConversion  OverrideOpt=off
  Sum : Sum  Inputs=+
  output_bus : Outport
  wires:
  Sum/1 -> Bus Creator/5  "numFeatures"
  Constant/1 -> Bus Creator/6  "mahal_dists"
  Signal Conversion/1 -> output_bus/1
  Bus Creator/1 -> Signal Conversion/1
  Compute Residual and H/4(R_mat) -> Bus Creator/4
  Compute Residual and H/3(H_out) -> Bus Creator/3
  Compute Residual and H/2(error_out) -> Bus Creator/2
  Compute Residual and H/1(r_out) -> Bus Creator/1
  vis_data/1 -> Bus Selector2/1
  Bus Selector2/1 -> [hr_observations], Compute Residual and H/6(O)  "<hr_observations>"
  Bus Selector3/2 -> [ml_quat_ISS2cam], Compute Residual and H/2(ml_quat_ISS2cam)  "<ml_quat_ISS2cam>"
  Bus Selector3/1 -> [ml_P_cam_ISS_ISS], Compute Residual and H/1(ml_P_cam_ISS_ISS)  "<ml_P_cam_ISS_ISS>"
  state_in/1 -> Bus Selector3/1
  aug_velocity/1 -> Bus Selector1/1
  Bus Selector1/1 -> Compute Residual and H/3(omega)  "<ml_vel_aug>"
  Bus Selector1/2 -> Compute Residual and H/4(velocity)  "<ml_omega_aug>"
  Bus Selector2/3 -> Compute Residual and H/9(hr_3d_knowledge_flag)  "<hr_3d_knowledge_flag>"
  Bus Selector2/4 -> Compute Global positions of Handrail Features/3(hr_P_hr_cam_cam)  "<hr_P_hr_cam_cam>"
  Bus Selector2/5 -> Compute Global positions of Handrail Features/4(hr_quat_cam2hr), [hr_quat_cam2hr]  "<hr_quat_cam2hr>"
  Bus Selector2/6 -> Compute Global positions of Handrail Features/7(hr_update_global_pose_flag)  "<hr_update_global_pose_flag>"
  Compute Global positions of Handrail Features/2(hr_P_hr_ISS_ISS) -> Bus Creator/7
  Compute Global positions of Handrail Features/3(hr_quat_ISS2hr) -> Bus Creator/8
  [ml_P_cam_ISS_ISS] -> Compute Global positions of Handrail Features/1(ml_P_cam_ISS_ISS)
  [ml_quat_ISS2cam] -> Compute Global positions of Handrail Features/2(ml_quat_ISS2cam)
  Bus Selector2/2 -> [hr_valid_flags], Compute Residual and H/7(valid)  "<hr_valid_flags>"
  [hr_observations] -> Compute Global positions of Handrail Features/5(hr_feature_observations)
  [hr_valid_flags] -> Compute Global positions of Handrail Features/6(hr_feature_valid)
  Compute Global positions of Handrail Features/1(hr_global_landmarks) -> [L]
  [L] -> Compute Residual and H/5(L)
  [hr_quat_cam2hr] -> Compute Residual and H/8(hr_quat_cam2hr)
  [hr_valid_flags] -> Data Type Conversion/1
  Data Type Conversion/1 -> Sum/1

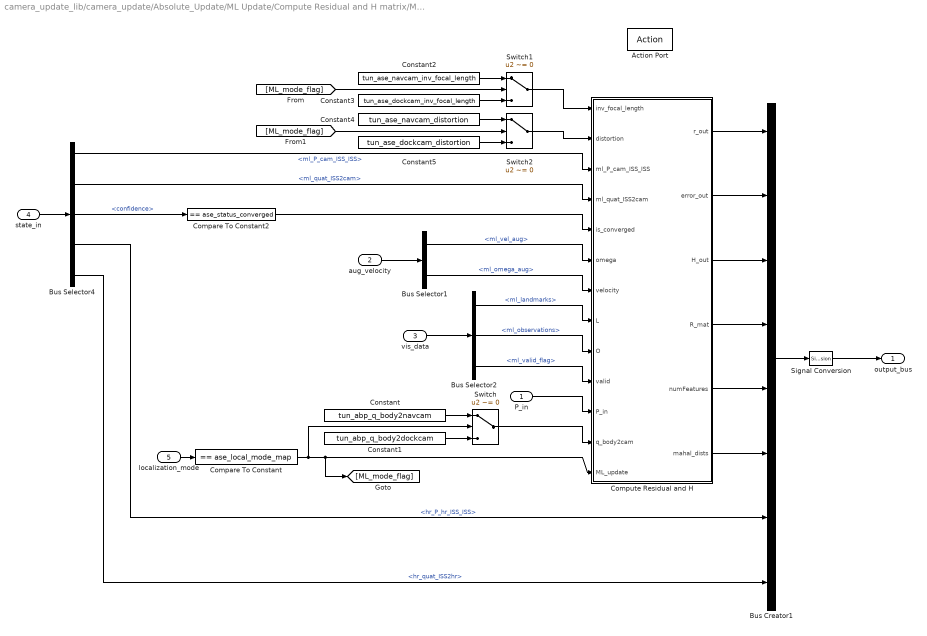
== system camera_update_lib/camera_update/Absolute_Update/ML Update/Compute Residual and H matrix/ML_Compute_Residual_and_H ==
  P_in : Inport
  aug_velocity : Inport  Port=2
  vis_data : Inport  Port=3
  state_in : Inport  Port=4
  localization_mode : Inport  Port=5
  Action Port : ActionPort
  Bus Creator1 : BusCreator  Inputs=8
  Bus Selector1 : BusSelector  OutputSignals=ml_vel_aug,ml_omega_aug
  Bus Selector2 : BusSelector  OutputSignals=ml_landmarks,ml_observations,ml_valid_flag
  Bus Selector4 : BusSelector  OutputSignals=ml_P_cam_ISS_ISS,ml_quat_ISS2cam,confidence,hr_P_hr_ISS_ISS,hr_quat_ISS2hr
  Compare To Constant : simulink/Logic and Bit Operations/Compare To Constant  relop===  const=ase_local_mode_map  OutDataTypeStr=boolean
  Compare To Constant2 : simulink/Logic and Bit Operations/Compare To Constant  relop===  const=ase_status_converged  OutDataTypeStr=boolean
  Compute Residual and H : MATLAB Function  TreatAsAtomicUnit=on
  Constant : Constant  Value=tun_abp_q_body2navcam
  Constant1 : Constant  Value=tun_abp_q_body2dockcam
  Constant2 : Constant  Value=tun_ase_navcam_inv_focal_length
  Constant3 : Constant  Value=tun_ase_dockcam_inv_focal_length
  Constant4 : Constant  Value=tun_ase_navcam_distortion
  Constant5 : Constant  Value=tun_ase_dockcam_distortion
  Signal Conversion : SignalConversion  OverrideOpt=off
  Switch : Switch  Criteria=u2 ~= 0
  Switch1 : Switch  Criteria=u2 ~= 0
  Switch2 : Switch  Criteria=u2 ~= 0
  output_bus : Outport
  wires:
  vis_data/1 -> Bus Selector2/1
  Bus Selector2/1 -> Compute Residual and H/8(L)  "<ml_landmarks>"
  Bus Selector2/2 -> Compute Residual and H/9(O)  "<ml_observations>"
  Bus Selector2/3 -> Compute Residual and H/10(valid)  "<ml_valid_flag>"
  Bus Selector4/3 -> Compare To Constant2/1  "<confidence>"
  Compare To Constant2/1 -> Compute Residual and H/5(is_converged)
  P_in/1 -> Compute Residual and H/11(P_in)
  Bus Selector4/2 -> Compute Residual and H/4(ml_quat_ISS2cam)  "<ml_quat_ISS2cam>"
  Bus Selector4/1 -> Compute Residual and H/3(ml_P_cam_ISS_ISS)  "<ml_P_cam_ISS_ISS>"
  aug_velocity/1 -> Bus Selector1/1
  Bus Selector1/1 -> Compute Residual and H/6(omega)  "<ml_vel_aug>"
  Bus Selector1/2 -> Compute Residual and H/7(velocity)  "<ml_omega_aug>"
  Compute Residual and H/2(error_out) -> Bus Creator1/2
  Compute Residual and H/6(mahal_dists) -> Bus Creator1/6
  Compute Residual and H/3(H_out) -> Bus Creator1/3
  Compute Residual and H/4(R_mat) -> Bus Creator1/4
  Compute Residual and H/5(numFeatures) -> Bus Creator1/5
  Compute Residual and H/1(r_out) -> Bus Creator1/1
  Bus Creator1/1 -> Signal Conversion/1
  Signal Conversion/1 -> output_bus/1
  localization_mode/1 -> Compare To Constant/1
  Compare To Constant/1 -> [ML_mode_flag], Compute Residual and H/13(ML_update), Switch/2
  Bus Selector4/5 -> Bus Creator1/8  "<hr_quat_ISS2hr>"
  Bus Selector4/4 -> Bus Creator1/7  "<hr_P_hr_ISS_ISS>"
  state_in/1 -> Bus Selector4/1
  Switch/1 -> Compute Residual and H/12(q_body2cam)
  Constant/1 -> Switch/1
  Constant1/1 -> Switch/3
  [ML_mode_flag] -> Switch1/2
  Constant2/1 -> Switch1/1
  Constant3/1 -> Switch1/3
  Switch1/1 -> Compute Residual and H/1(inv_focal_length)
  [ML_mode_flag] -> Switch2/2
  Constant4/1 -> Switch2/1
  Constant5/1 -> Switch2/3
  Switch2/1 -> Compute Residual and H/2(distortion)

== system camera_update_lib/camera_update/Absolute_Update/ML Update/ML_correector/apply_delta_state ==
  kfl_msg_in : Inport
  delta_state_in : Inport  Port=2
  Bus Assignment1 : BusAssignment  AssignedSignals=quat_ISS2B,gyro_bias,V_B_ISS_ISS,accel_bias,P_EST_ISS_ISS,ml_quat_ISS2cam,ml_P_cam_ISS_ISS,kfl_status,of_quat_ISS2cam,of_P_cam_ISS_ISS
  Bus Selector1 : BusSelector  OutputSignals=quat_ISS2B,gyro_bias,V_B_ISS_ISS,accel_bias,P_EST_ISS_ISS,ml_quat_ISS2cam,ml_P_cam_ISS_ISS,kfl_status,of_quat_ISS2cam,of_P_cam_ISS_ISS
  Constant : Constant  Value=uint16(1)
  ex_apply_delta_state : S-Function  FunctionName=ex_apply_delta_state  SFunctionDeploymentMode=off  EnableBusSupport=off  mask(Legacy Function){SFunctionSpec=void apply_delta_state(single u1[], int32 size(u1, 1), uint16 u2, single u3[4], single u4[3], single u5[3], single u6[3], single u7[3], single u8[4], single u9[3], uint16 u10, single u11[16][4], single u12[16][3], single y1[4], single y2[3], single y3[3], single y4[3], single y5[3], single y6[4], single y7[3], uint16 y8[1], single y9[16][4], single y10[16][3]), ShowSpec=off}
      mask prompts: ShowSpec "Display function specification"
      mask help:
      | This block allows you to call the legacy functions specified by the following Legacy Code Tool definition:
      | def.SFunctionName = 'ex_apply_delta_state';
      | def.OutputFcnSpec = 'void apply_delta_state(single u1[], int32 size(u1, 1), uint16 u2, single u3[4], single u4[3], single u5[3], single u6[3], single u7[3], single u8[4], single u9[3], uint16 u10, single u11[16][4], single u12[16][3], single y1[4], single y2[3], single y3[3], single y4[3], single y5[3], single y6[4], single y7[3], uint16 y8[1], single y9[16][4], single y10[16][3])';
      | def.HeaderFiles = {'apply_delta_state.h'};
      | def.SourceFiles = {'apply_delta_state.cpp'};
      | def.IncPaths = {'cxx_functions/include', '/usr/include/eigen3'};
      | def.SrcPaths = {'cxx_functions/src', '/usr/include/eigen3/Eigen/src'};
      | def.Options.language = 'C++';
      mask Help: <p>This block was generated automatically by the Legacy Code Tool. For detailed help on this tool, call<a href="matlab:legacy_code('help')"> legacy_code('help')</a>.</p>
      mask Callback ShowSpec:
      | if strcmp(get_param(gcbh, 'ShowSpec'), 'on')
      |   set_param(gcbh, 'MaskDisplay', sprintf('fprintf(''%s'');', get_param(gcbh, 'SFunctionSpec')));
      | else
      |   set_param(gcbh, 'MaskDisplay', sprintf('fprintf(''%s'');', get_param(gcbh, 'FunctionName')));
      | end
      mask Display: fprintf('ex_apply_delta_state');
  kfl_msg_out : Outport
  wires:
  ex_apply_delta_state/10 -> Bus Assignment1/11
  ex_apply_delta_state/8 -> Bus Assignment1/9
  ex_apply_delta_state/7 -> Bus Assignment1/8
  ex_apply_delta_state/5 -> Bus Assignment1/6
  ex_apply_delta_state/4 -> Bus Assignment1/5
  ex_apply_delta_state/3 -> Bus Assignment1/4
  ex_apply_delta_state/2 -> Bus Assignment1/3
  Bus Selector1/10 -> ex_apply_delta_state/12  "<of_P_cam_ISS_ISS>"
  Bus Selector1/9 -> ex_apply_delta_state/11  "<of_quat_ISS2cam>"
  Bus Selector1/8 -> ex_apply_delta_state/10  "<kfl_status>"
  Bus Selector1/7 -> ex_apply_delta_state/9  "<ml_P_cam_ISS_ISS>"
  Bus Selector1/6 -> ex_apply_delta_state/8  "<ml_quat_ISS2cam>"
  Bus Selector1/5 -> ex_apply_delta_state/7  "<P_EST_ISS_ISS>"
  Bus Selector1/4 -> ex_apply_delta_state/6  "<accel_bias>"
  Bus Selector1/3 -> ex_apply_delta_state/5  "<V_B_ISS_ISS>"
  Bus Selector1/2 -> ex_apply_delta_state/4  "<gyro_bias>"
  Bus Selector1/1 -> ex_apply_delta_state/3  "<quat_ISS2B>"
  Constant/1 -> ex_apply_delta_state/2
  delta_state_in/1 -> ex_apply_delta_state/1
  kfl_msg_in/1 -> Bus Assignment1/1, Bus Selector1/1
  Bus Assignment1/1 -> kfl_msg_out/1
  ex_apply_delta_state/1 -> Bus Assignment1/2
  ex_apply_delta_state/9 -> Bus Assignment1/10
  ex_apply_delta_state/6 -> Bus Assignment1/7

== matlab function camera_update_lib/camera_update/Absolute_Update/ML Update/Compute Residual and H matrix/HR_Compute_Residual_and_H1/Compute Global positions of Handrail Features ==
  data: ml_P_cam_ISS_ISS input; ml_quat_ISS2cam input; hr_P_hr_cam_cam input; hr_quat_cam2hr input; hr_feature_observations input; hr_feature_valid input; hr_update_global_pose_flag input; hr_global_landmarks output; hr_P_hr_ISS_ISS output; hr_quat_ISS2hr output
function [hr_global_landmarks, hr_P_hr_ISS_ISS, hr_quat_ISS2hr]  = compute_hr_tf_and_landmark(ml_P_cam_ISS_ISS, ml_quat_ISS2cam, hr_P_hr_cam_cam, hr_quat_cam2hr, ...
                                       hr_feature_observations, hr_feature_valid, hr_update_global_pose_flag)        
                                     
[hr_global_landmarks, hr_P_hr_ISS_ISS, hr_quat_ISS2hr] = compute_hr_tf_and_landmark(ml_P_cam_ISS_ISS, ml_quat_ISS2cam, hr_P_hr_cam_cam, hr_quat_cam2hr, ...
                                       hr_feature_observations, hr_feature_valid, hr_update_global_pose_flag);

== matlab function camera_update_lib/camera_update/Optical_Flow_Update/OF Update/Compute_DeltaState_and_Covariance ==
  data: error_out output; residual input; H input; R_mat input; P input; delta_state output size=ase_total_num_states; P_out output ase_cov_datatype size=[ase_total_num_states ase_total_num_states]
% Calculate the delta State
function [error_out, delta_state, P_out]  = HPH(residual, H, R_mat, P)
%#codegen
[error_out, delta_state, P_out]  = eml_compute_delta_state_and_cov(residual, 0, H, R_mat, P);

== matlab function camera_update_lib/camera_update/Optical_Flow_Update/OF Update/Simulink Compute H and R/compute_of_residual_and_h ==
  data: error_out output; of_measured input size=2 * ase_of_num_aug * cvs_optflow_num_out; r output size=[(2*ase_of_num_aug-3)*ase_of_num_features 1]; H output size=[(2*ase_of_num_aug-3)*ase_of_num_features ase_total_num_states]; global_points input size=[4 cvs_optflow_num_out]; camera_tf_global input; valid input; num_of_tracks output; ase_of_num_aug parameter; mahal_dists output size=ase_of_num_features; ase_of_num_features parameter; tun_ase_mahal_distance_max parameter; tun_ase_of_r_mag parameter; P input
% Code is taken from Zack Morrato's prototyped Optical Flow Kalman Filter.
% This code computes the residual and measurment matrices for the optical
% flow measurments.
%
%
function [ error_out, r, H, num_of_tracks, mahal_dists ] = compute_of_residual_and_h(of_measured, global_points, camera_tf_global, valid, ase_of_num_aug, ase_of_num_features, tun_ase_mahal_distance_max, tun_ase_of_r_mag,  P)
%#codegen
[ r, H, error_out, num_of_tracks, mahal_dists] = eml_compute_of_residual_and_h(of_measured, global_points, camera_tf_global, valid, ase_of_num_aug, ase_of_num_features, tun_ase_mahal_distance_max, tun_ase_of_r_mag, P);

== matlab function camera_update_lib/camera_update/Optical_Flow_Update/OF Update/compute_of_global_points ==
  data: of_measured output size=2 * ase_of_num_aug * ase_of_num_features; global_points output size=[4 ase_of_num_features]; of_quat_ISS2CAM input; of_P_cam_ISS_ISS input; of_measured_in input; valid input; tun_ase_vocam_inv_focal_length parameter; camera_tf_global output size=[ase_of_num_aug*4 4]; ase_of_num_aug parameter; valid_out output size=[ase_of_num_features ase_of_num_aug]; num_of_tracks output
% Code is taken from Zack Morrato's prototyped Optical Flow Kalman Filter.
% This code computes the residual and measurment matrices for the optical
% flow measurments.
%
%
function [of_measured, global_points, camera_tf_global, valid_out, num_of_tracks]   = compute_of_global_points(of_quat_ISS2CAM, of_P_cam_ISS_ISS, of_measured_in, valid, tun_ase_vocam_inv_focal_length, ase_of_num_aug)
%#codegen
[of_measured, global_points, camera_tf_global, valid_out, num_of_tracks] = eml_compute_of_global_points(of_quat_ISS2CAM, of_P_cam_ISS_ISS, of_measured_in, valid, tun_ase_vocam_inv_focal_length, ase_of_num_aug);

== matlab function camera_update_lib/camera_update/Optical_Flow_Update/OF Update/Simulink Compute H and R/compress_of_residual_and_h ==
  data: r input size=[(2*ase_of_num_aug-3)*cvs_optflow_num_out 1]; r_comp output size=[6*ase_of_num_aug 1]; H_comp output size=[6*ase_of_num_aug ase_total_num_states]; H input size=[(2*ase_of_num_aug-3)*cvs_optflow_num_out ase_total_num_states]; ase_of_num_aug parameter
% Code is taken from Zack Morrato's prototyped Optical Flow Kalman Filter.
% This code computes the residual and measurment matrices for the optical
% flow measurments.
%
%
function [ r_comp, H_comp] = compress_of_residual_and_h(r, H, ase_of_num_aug)
%#codegen
[ r_comp, H_comp] = eml_of_residual_and_h_compress(r, H, ase_of_num_aug);

== matlab function camera_update_lib/camera_update/Absolute_Update/ML Update/Compute Residual and H matrix/HR_Compute_Residual_and_H1/Compute Residual and H ==
  data: ml_P_cam_ISS_ISS input; ml_quat_ISS2cam input; omega input size=3; velocity input size=3; L input; O input; valid input; ase_of_num_aug parameter; ase_hr_r_mag parameter; ase_hr_distance_r parameter; tun_abp_q_body2perchcam parameter; tun_ase_ml_forward_projection_time parameter; r_out output size=[6 1]; error_out output; H_out output size=[6 ase_total_num_states]; R_mat output size=[6 6]; hr_quat_cam2hr input; hr_3d_knowledge_flag input
function [r_out, error_out, H_out, R_mat] = eml_compute_hr_residual_and_h(ml_P_cam_ISS_ISS, ml_quat_ISS2cam, omega, velocity, L, O, valid, ase_of_num_aug, ase_hr_r_mag, ase_hr_distance_r, tun_abp_q_body2perchcam, tun_ase_ml_forward_projection_time, hr_quat_cam2hr,hr_3d_knowledge_flag)
%#codegen
[r_out, error_out, H_out, R_mat] = eml_compute_hr_residual_and_h(ml_P_cam_ISS_ISS, ml_quat_ISS2cam, omega, velocity, L, O, valid, ase_of_num_aug, ase_hr_r_mag, ase_hr_distance_r, tun_ase_ml_forward_projection_time, tun_abp_q_body2perchcam, hr_quat_cam2hr, hr_3d_knowledge_flag);
